simulink model "TST_RailP_VDGradMon"  (R2016b)
settings: Solver=FixedStepDiscrete  StartTime=0.0  StopTime=simTime  FixedStep=sampleTime  RelTol=1e-3
values from neighbouring files (symbols this model uses):
  testCase = 1    [initTST_RailP_VDGradMon_001.m]    (also in initTST_RailP_VDGradMon_002.m = 2; initTST_RailP_VDGradMon_003.m = 3; initTST_RailP_VDGradMon_004.m = 4; initTST_RailP_VDGradMon_005.m = 5)
libraries: simulink x6
settings Model: Creator=wolf072601  LastModifiedBy=wolf072601
settings DebuggingCC: SignalRangeChecking=error

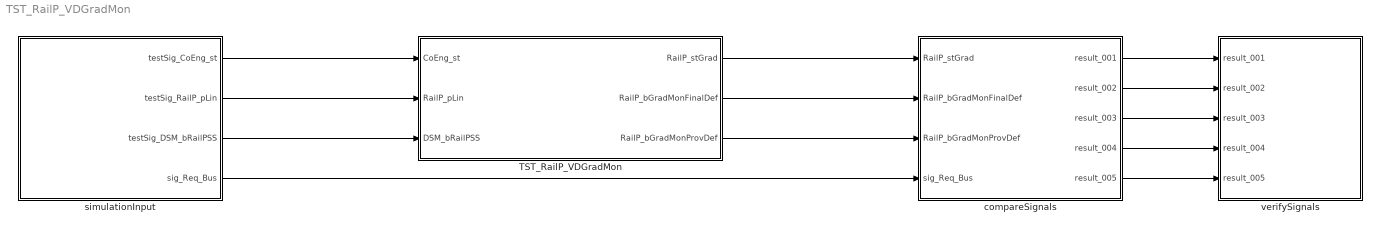
== system TST_RailP_VDGradMon ==
  TST_RailP_VDGradMon : Subsystem
  compareSignals : Subsystem
  simulationInput : Subsystem
  verifySignals : Subsystem
  wires:
  simulationInput/1(testSig_CoEng_st) -> TST_RailP_VDGradMon/1(CoEng_st)
  simulationInput/2(testSig_RailP_pLin) -> TST_RailP_VDGradMon/2(RailP_pLin)
  simulationInput/3(testSig_DSM_bRailPSS) -> TST_RailP_VDGradMon/3(DSM_bRailPSS)
  TST_RailP_VDGradMon/1(RailP_stGrad) -> compareSignals/1(RailP_stGrad)
  TST_RailP_VDGradMon/2(RailP_bGradMonFinalDef) -> compareSignals/2(RailP_bGradMonFinalDef)
  TST_RailP_VDGradMon/3(RailP_bGradMonProvDef) -> compareSignals/3(RailP_bGradMonProvDef)
  simulationInput/4(sig_Req_Bus) -> compareSignals/4(sig_Req_Bus)
  compareSignals/1(result_001) -> verifySignals/1(result_001)
  compareSignals/2(result_002) -> verifySignals/2(result_002)
  compareSignals/3(result_003) -> verifySignals/3(result_003)
  compareSignals/4(result_004) -> verifySignals/4(result_004)
  compareSignals/5(result_005) -> verifySignals/5(result_005)

== system TST_RailP_VDGradMon/TST_RailP_VDGradMon ==
  CoEng_st : Inport
  RailP_pLin : Inport  Port=2
  DSM_bRailPSS : Inport  Port=3
  Function_Call : simulink/Ports & Subsystems/Function-Call Generator  sample_time=sampleTime  numberOfIterations=1
  RailP_VDGradMon : ModelReference  ModelNameDialog=RailP_VDGradMon  ModelReferenceVersion=1.19  TriggerPortName=function  TriggerPortTriggerType=function-call  TriggerPortStatesWhenEnabling=held
  RailP_stGrad : Outport
  RailP_bGradMonFinalDef : Outport  Port=2
  RailP_bGradMonProvDef : Outport  Port=3
  wires:
  Function_Call/1 -> RailP_VDGradMon/Trigger
  CoEng_st/1 -> RailP_VDGradMon/1
  RailP_pLin/1 -> RailP_VDGradMon/2
  DSM_bRailPSS/1 -> RailP_VDGradMon/3
  RailP_VDGradMon/1 -> RailP_stGrad/1
  RailP_VDGradMon/2 -> RailP_bGradMonFinalDef/1
  RailP_VDGradMon/3 -> RailP_bGradMonProvDef/1

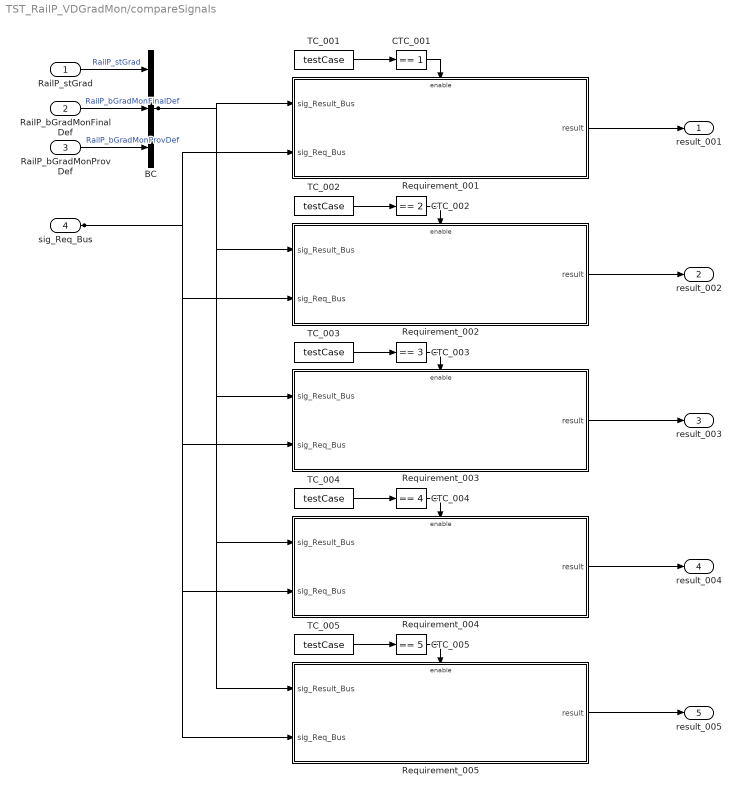
== system TST_RailP_VDGradMon/compareSignals ==
  RailP_stGrad : Inport
  RailP_bGradMonFinalDef : Inport  Port=2
  RailP_bGradMonProvDef : Inport  Port=3
  sig_Req_Bus : Inport  Port=4
  BC : BusCreator  Inputs=3
  CTC_001 : simulink/Logic and Bit Operations/Compare To Constant  relop===  const=1  OutDataTypeStr=boolean
  CTC_002 : simulink/Logic and Bit Operations/Compare To Constant  relop===  const=2  OutDataTypeStr=boolean
  CTC_003 : simulink/Logic and Bit Operations/Compare To Constant  relop===  const=3  OutDataTypeStr=boolean
  CTC_004 : simulink/Logic and Bit Operations/Compare To Constant  relop===  const=4  OutDataTypeStr=boolean
  CTC_005 : simulink/Logic and Bit Operations/Compare To Constant  relop===  const=5  OutDataTypeStr=boolean
  Requirement_001 : Subsystem
  Requirement_002 : Subsystem
  Requirement_003 : Subsystem
  Requirement_004 : Subsystem
  Requirement_005 : Subsystem
  TC_001 : Constant  Value=testCase
  TC_002 : Constant  Value=testCase
  TC_003 : Constant  Value=testCase
  TC_004 : Constant  Value=testCase
  TC_005 : Constant  Value=testCase
  result_001 : Outport
  result_002 : Outport  Port=2
  result_003 : Outport  Port=3
  result_004 : Outport  Port=4
  result_005 : Outport  Port=5
  wires:
  RailP_stGrad/1 -> BC/1  "RailP_stGrad"
  RailP_bGradMonFinalDef/1 -> BC/2  "RailP_bGradMonFinalDef"
  RailP_bGradMonProvDef/1 -> BC/3  "RailP_bGradMonProvDef"
  TC_001/1 -> CTC_001/1
  CTC_001/1 -> Requirement_001/Enable
  sig_Req_Bus/1 -> Requirement_001/2(sig_Req_Bus), Requirement_002/2(sig_Req_Bus), Requirement_003/2(sig_Req_Bus), Requirement_004/2(sig_Req_Bus), Requirement_005/2(sig_Req_Bus)
  BC/1 -> Requirement_001/1(sig_Result_Bus), Requirement_002/1(sig_Result_Bus), Requirement_003/1(sig_Result_Bus), Requirement_004/1(sig_Result_Bus), Requirement_005/1(sig_Result_Bus)
  Requirement_001/1(result) -> result_001/1
  TC_002/1 -> CTC_002/1
  CTC_002/1 -> Requirement_002/Enable
  Requirement_002/1(result) -> result_002/1
  TC_003/1 -> CTC_003/1
  CTC_003/1 -> Requirement_003/Enable
  Requirement_003/1(result) -> result_003/1
  TC_004/1 -> CTC_004/1
  CTC_004/1 -> Requirement_004/Enable
  Requirement_004/1(result) -> result_004/1
  TC_005/1 -> CTC_005/1
  CTC_005/1 -> Requirement_005/Enable
  Requirement_005/1(result) -> result_005/1

== system TST_RailP_VDGradMon/simulationInput ==
  BS : BusSelector  OutputSignals=testSig_CoEng_st,testSig_RailP_pLin,testSig_DSM_bRailPSS
  MPSw : MultiPortSwitch  Inputs=5  SaturateOnIntegerOverflow=on  InputSameDT=on
  TestCase : Constant  Value=testCase
  testSignals_R001 : Subsystem
  testSignals_R002 : Subsystem
  testSignals_R003 : Subsystem
  testSignals_R004 : Subsystem
  testSignals_R005 : Subsystem
  testSig_CoEng_st : Outport
  testSig_RailP_pLin : Outport  Port=2
  testSig_DSM_bRailPSS : Outport  Port=3
  sig_Req_Bus : Outport  Port=4
  wires:
  BS/1 -> testSig_CoEng_st/1  "<testSig_CoEng_st>"
  BS/2 -> testSig_RailP_pLin/1  "<testSig_RailP_pLin>"
  BS/3 -> testSig_DSM_bRailPSS/1  "<testSig_DSM_bRailPSS>"
  MPSw/1 -> BS/1, sig_Req_Bus/1
  TestCase/1 -> MPSw/1
  testSignals_R001/1(testSignals) -> MPSw/2
  testSignals_R002/1(testSignals) -> MPSw/3
  testSignals_R003/1(testSignals) -> MPSw/4
  testSignals_R004/1(testSignals) -> MPSw/5
  testSignals_R005/1(testSignals) -> MPSw/6

== system TST_RailP_VDGradMon/verifySignals ==
  result_001 : Inport
  result_002 : Inport  Port=2
  result_003 : Inport  Port=3
  result_004 : Inport  Port=4
  result_005 : Inport  Port=5
  Assertion_001 : Assertion  Enabled=off
  Assertion_002 : Assertion  Enabled=off
  Assertion_003 : Assertion  Enabled=off
  Assertion_004 : Assertion  Enabled=off
  Assertion_005 : Assertion  Enabled=off
  wires:
  result_001/1 -> Assertion_001/1
  result_002/1 -> Assertion_002/1
  result_003/1 -> Assertion_003/1
  result_004/1 -> Assertion_004/1
  result_005/1 -> Assertion_005/1

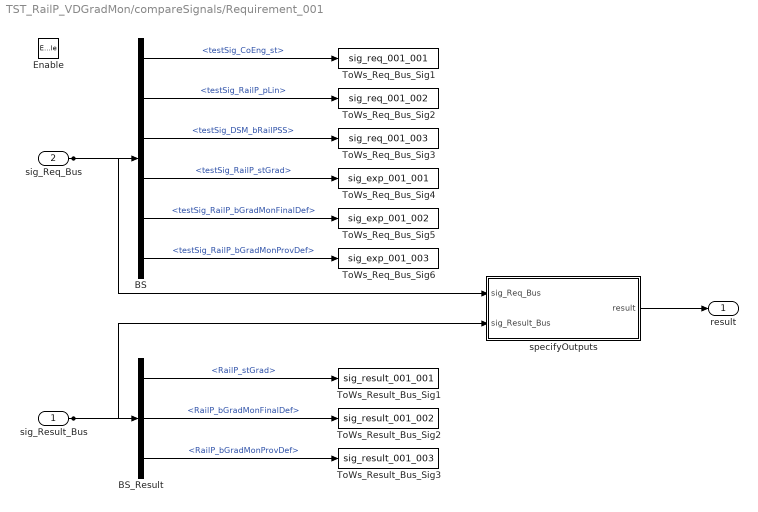
== system TST_RailP_VDGradMon/compareSignals/Requirement_001 ==
  sig_Result_Bus : Inport
  sig_Req_Bus : Inport  Port=2
  Enable : EnablePort
  BS : BusSelector  OutputSignals=testSig_CoEng_st,testSig_RailP_pLin,testSig_DSM_bRailPSS,testSig_RailP_stGrad,testSig_RailP_bGradMonFinalDef,testSig_RailP_bGradMonProvDef
  BS_Result : BusSelector  OutputSignals=RailP_stGrad,RailP_bGradMonFinalDef,RailP_bGradMonProvDef
  ToWs_Req_Bus_Sig1 : ToWorkspace  VariableName=sig_req_001_001  SaveFormat=Structure With Time
  ToWs_Req_Bus_Sig2 : ToWorkspace  VariableName=sig_req_001_002  SaveFormat=Structure With Time
  ToWs_Req_Bus_Sig3 : ToWorkspace  VariableName=sig_req_001_003  SaveFormat=Structure With Time
  ToWs_Req_Bus_Sig4 : ToWorkspace  VariableName=sig_exp_001_001  SaveFormat=Structure With Time
  ToWs_Req_Bus_Sig5 : ToWorkspace  VariableName=sig_exp_001_002  SaveFormat=Structure With Time
  ToWs_Req_Bus_Sig6 : ToWorkspace  VariableName=sig_exp_001_003  SaveFormat=Structure With Time
  ToWs_Result_Bus_Sig1 : ToWorkspace  VariableName=sig_result_001_001  SaveFormat=Structure With Time
  ToWs_Result_Bus_Sig2 : ToWorkspace  VariableName=sig_result_001_002  SaveFormat=Structure With Time
  ToWs_Result_Bus_Sig3 : ToWorkspace  VariableName=sig_result_001_003  SaveFormat=Structure With Time
  specifyOutputs : Subsystem
  result : Outport
  wires:
  sig_Req_Bus/1 -> BS/1, specifyOutputs/1(sig_Req_Bus)
  BS/1 -> ToWs_Req_Bus_Sig1/1  "<testSig_CoEng_st>"
  BS/2 -> ToWs_Req_Bus_Sig2/1  "<testSig_RailP_pLin>"
  BS/3 -> ToWs_Req_Bus_Sig3/1  "<testSig_DSM_bRailPSS>"
  BS/4 -> ToWs_Req_Bus_Sig4/1  "<testSig_RailP_stGrad>"
  BS/5 -> ToWs_Req_Bus_Sig5/1  "<testSig_RailP_bGradMonFinalDef>"
  BS/6 -> ToWs_Req_Bus_Sig6/1  "<testSig_RailP_bGradMonProvDef>"
  sig_Result_Bus/1 -> BS_Result/1, specifyOutputs/2(sig_Result_Bus)
  BS_Result/1 -> ToWs_Result_Bus_Sig1/1  "<RailP_stGrad>"
  BS_Result/2 -> ToWs_Result_Bus_Sig2/1  "<RailP_bGradMonFinalDef>"
  BS_Result/3 -> ToWs_Result_Bus_Sig3/1  "<RailP_bGradMonProvDef>"
  specifyOutputs/1(result) -> result/1

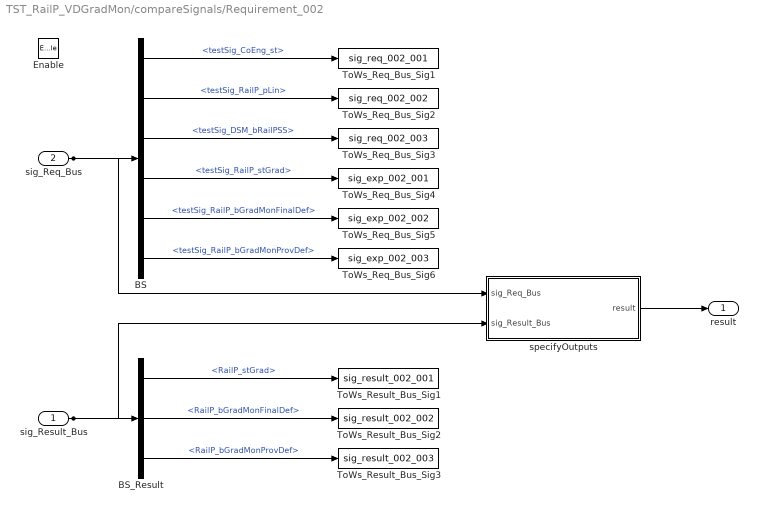
== system TST_RailP_VDGradMon/compareSignals/Requirement_002 ==
  sig_Result_Bus : Inport
  sig_Req_Bus : Inport  Port=2
  Enable : EnablePort
  BS : BusSelector  OutputSignals=testSig_CoEng_st,testSig_RailP_pLin,testSig_DSM_bRailPSS,testSig_RailP_stGrad,testSig_RailP_bGradMonFinalDef,testSig_RailP_bGradMonProvDef
  BS_Result : BusSelector  OutputSignals=RailP_stGrad,RailP_bGradMonFinalDef,RailP_bGradMonProvDef
  ToWs_Req_Bus_Sig1 : ToWorkspace  VariableName=sig_req_002_001  SaveFormat=Structure With Time
  ToWs_Req_Bus_Sig2 : ToWorkspace  VariableName=sig_req_002_002  SaveFormat=Structure With Time
  ToWs_Req_Bus_Sig3 : ToWorkspace  VariableName=sig_req_002_003  SaveFormat=Structure With Time
  ToWs_Req_Bus_Sig4 : ToWorkspace  VariableName=sig_exp_002_001  SaveFormat=Structure With Time
  ToWs_Req_Bus_Sig5 : ToWorkspace  VariableName=sig_exp_002_002  SaveFormat=Structure With Time
  ToWs_Req_Bus_Sig6 : ToWorkspace  VariableName=sig_exp_002_003  SaveFormat=Structure With Time
  ToWs_Result_Bus_Sig1 : ToWorkspace  VariableName=sig_result_002_001  SaveFormat=Structure With Time
  ToWs_Result_Bus_Sig2 : ToWorkspace  VariableName=sig_result_002_002  SaveFormat=Structure With Time
  ToWs_Result_Bus_Sig3 : ToWorkspace  VariableName=sig_result_002_003  SaveFormat=Structure With Time
  specifyOutputs : Subsystem
  result : Outport
  wires:
  sig_Req_Bus/1 -> BS/1, specifyOutputs/1(sig_Req_Bus)
  BS/1 -> ToWs_Req_Bus_Sig1/1  "<testSig_CoEng_st>"
  BS/2 -> ToWs_Req_Bus_Sig2/1  "<testSig_RailP_pLin>"
  BS/3 -> ToWs_Req_Bus_Sig3/1  "<testSig_DSM_bRailPSS>"
  BS/4 -> ToWs_Req_Bus_Sig4/1  "<testSig_RailP_stGrad>"
  BS/5 -> ToWs_Req_Bus_Sig5/1  "<testSig_RailP_bGradMonFinalDef>"
  BS/6 -> ToWs_Req_Bus_Sig6/1  "<testSig_RailP_bGradMonProvDef>"
  sig_Result_Bus/1 -> BS_Result/1, specifyOutputs/2(sig_Result_Bus)
  BS_Result/1 -> ToWs_Result_Bus_Sig1/1  "<RailP_stGrad>"
  BS_Result/2 -> ToWs_Result_Bus_Sig2/1  "<RailP_bGradMonFinalDef>"
  BS_Result/3 -> ToWs_Result_Bus_Sig3/1  "<RailP_bGradMonProvDef>"
  specifyOutputs/1(result) -> result/1

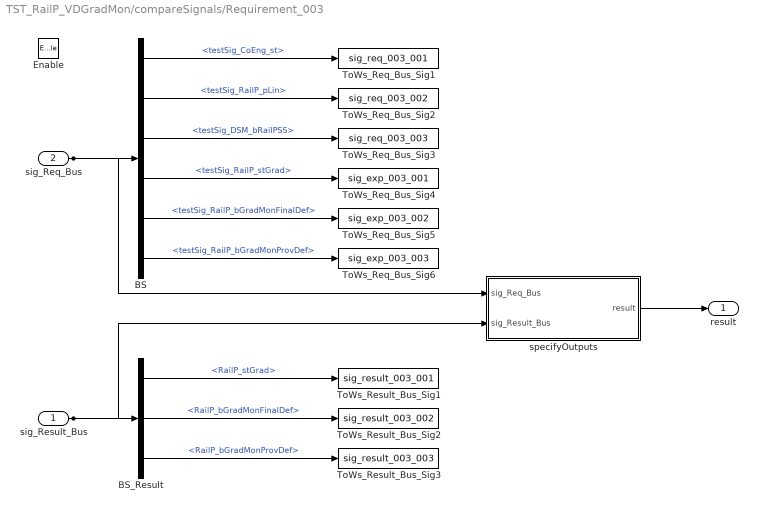
== system TST_RailP_VDGradMon/compareSignals/Requirement_003 ==
  sig_Result_Bus : Inport
  sig_Req_Bus : Inport  Port=2
  Enable : EnablePort
  BS : BusSelector  OutputSignals=testSig_CoEng_st,testSig_RailP_pLin,testSig_DSM_bRailPSS,testSig_RailP_stGrad,testSig_RailP_bGradMonFinalDef,testSig_RailP_bGradMonProvDef
  BS_Result : BusSelector  OutputSignals=RailP_stGrad,RailP_bGradMonFinalDef,RailP_bGradMonProvDef
  ToWs_Req_Bus_Sig1 : ToWorkspace  VariableName=sig_req_003_001  SaveFormat=Structure With Time
  ToWs_Req_Bus_Sig2 : ToWorkspace  VariableName=sig_req_003_002  SaveFormat=Structure With Time
  ToWs_Req_Bus_Sig3 : ToWorkspace  VariableName=sig_req_003_003  SaveFormat=Structure With Time
  ToWs_Req_Bus_Sig4 : ToWorkspace  VariableName=sig_exp_003_001  SaveFormat=Structure With Time
  ToWs_Req_Bus_Sig5 : ToWorkspace  VariableName=sig_exp_003_002  SaveFormat=Structure With Time
  ToWs_Req_Bus_Sig6 : ToWorkspace  VariableName=sig_exp_003_003  SaveFormat=Structure With Time
  ToWs_Result_Bus_Sig1 : ToWorkspace  VariableName=sig_result_003_001  SaveFormat=Structure With Time
  ToWs_Result_Bus_Sig2 : ToWorkspace  VariableName=sig_result_003_002  SaveFormat=Structure With Time
  ToWs_Result_Bus_Sig3 : ToWorkspace  VariableName=sig_result_003_003  SaveFormat=Structure With Time
  specifyOutputs : Subsystem
  result : Outport
  wires:
  sig_Req_Bus/1 -> BS/1, specifyOutputs/1(sig_Req_Bus)
  BS/1 -> ToWs_Req_Bus_Sig1/1  "<testSig_CoEng_st>"
  BS/2 -> ToWs_Req_Bus_Sig2/1  "<testSig_RailP_pLin>"
  BS/3 -> ToWs_Req_Bus_Sig3/1  "<testSig_DSM_bRailPSS>"
  BS/4 -> ToWs_Req_Bus_Sig4/1  "<testSig_RailP_stGrad>"
  BS/5 -> ToWs_Req_Bus_Sig5/1  "<testSig_RailP_bGradMonFinalDef>"
  BS/6 -> ToWs_Req_Bus_Sig6/1  "<testSig_RailP_bGradMonProvDef>"
  sig_Result_Bus/1 -> BS_Result/1, specifyOutputs/2(sig_Result_Bus)
  BS_Result/1 -> ToWs_Result_Bus_Sig1/1  "<RailP_stGrad>"
  BS_Result/2 -> ToWs_Result_Bus_Sig2/1  "<RailP_bGradMonFinalDef>"
  BS_Result/3 -> ToWs_Result_Bus_Sig3/1  "<RailP_bGradMonProvDef>"
  specifyOutputs/1(result) -> result/1

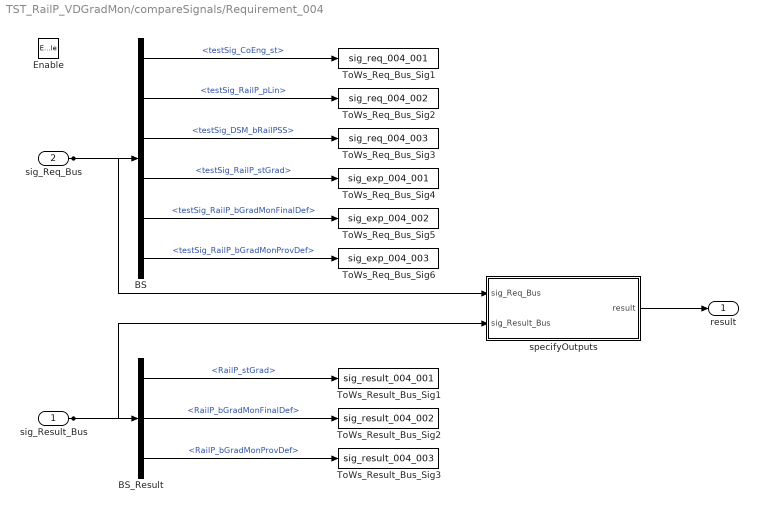
== system TST_RailP_VDGradMon/compareSignals/Requirement_004 ==
  sig_Result_Bus : Inport
  sig_Req_Bus : Inport  Port=2
  Enable : EnablePort
  BS : BusSelector  OutputSignals=testSig_CoEng_st,testSig_RailP_pLin,testSig_DSM_bRailPSS,testSig_RailP_stGrad,testSig_RailP_bGradMonFinalDef,testSig_RailP_bGradMonProvDef
  BS_Result : BusSelector  OutputSignals=RailP_stGrad,RailP_bGradMonFinalDef,RailP_bGradMonProvDef
  ToWs_Req_Bus_Sig1 : ToWorkspace  VariableName=sig_req_004_001  SaveFormat=Structure With Time
  ToWs_Req_Bus_Sig2 : ToWorkspace  VariableName=sig_req_004_002  SaveFormat=Structure With Time
  ToWs_Req_Bus_Sig3 : ToWorkspace  VariableName=sig_req_004_003  SaveFormat=Structure With Time
  ToWs_Req_Bus_Sig4 : ToWorkspace  VariableName=sig_exp_004_001  SaveFormat=Structure With Time
  ToWs_Req_Bus_Sig5 : ToWorkspace  VariableName=sig_exp_004_002  SaveFormat=Structure With Time
  ToWs_Req_Bus_Sig6 : ToWorkspace  VariableName=sig_exp_004_003  SaveFormat=Structure With Time
  ToWs_Result_Bus_Sig1 : ToWorkspace  VariableName=sig_result_004_001  SaveFormat=Structure With Time
  ToWs_Result_Bus_Sig2 : ToWorkspace  VariableName=sig_result_004_002  SaveFormat=Structure With Time
  ToWs_Result_Bus_Sig3 : ToWorkspace  VariableName=sig_result_004_003  SaveFormat=Structure With Time
  specifyOutputs : Subsystem
  result : Outport
  wires:
  sig_Req_Bus/1 -> BS/1, specifyOutputs/1(sig_Req_Bus)
  BS/1 -> ToWs_Req_Bus_Sig1/1  "<testSig_CoEng_st>"
  BS/2 -> ToWs_Req_Bus_Sig2/1  "<testSig_RailP_pLin>"
  BS/3 -> ToWs_Req_Bus_Sig3/1  "<testSig_DSM_bRailPSS>"
  BS/4 -> ToWs_Req_Bus_Sig4/1  "<testSig_RailP_stGrad>"
  BS/5 -> ToWs_Req_Bus_Sig5/1  "<testSig_RailP_bGradMonFinalDef>"
  BS/6 -> ToWs_Req_Bus_Sig6/1  "<testSig_RailP_bGradMonProvDef>"
  sig_Result_Bus/1 -> BS_Result/1, specifyOutputs/2(sig_Result_Bus)
  BS_Result/1 -> ToWs_Result_Bus_Sig1/1  "<RailP_stGrad>"
  BS_Result/2 -> ToWs_Result_Bus_Sig2/1  "<RailP_bGradMonFinalDef>"
  BS_Result/3 -> ToWs_Result_Bus_Sig3/1  "<RailP_bGradMonProvDef>"
  specifyOutputs/1(result) -> result/1

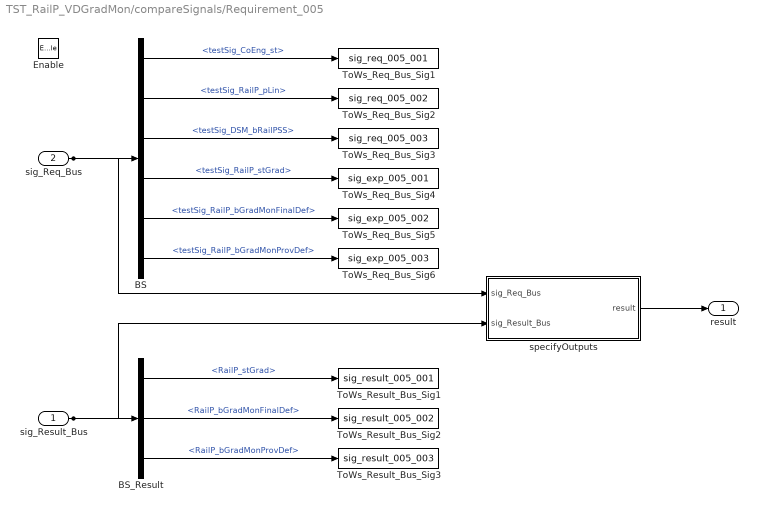
== system TST_RailP_VDGradMon/compareSignals/Requirement_005 ==
  sig_Result_Bus : Inport
  sig_Req_Bus : Inport  Port=2
  Enable : EnablePort
  BS : BusSelector  OutputSignals=testSig_CoEng_st,testSig_RailP_pLin,testSig_DSM_bRailPSS,testSig_RailP_stGrad,testSig_RailP_bGradMonFinalDef,testSig_RailP_bGradMonProvDef
  BS_Result : BusSelector  OutputSignals=RailP_stGrad,RailP_bGradMonFinalDef,RailP_bGradMonProvDef
  ToWs_Req_Bus_Sig1 : ToWorkspace  VariableName=sig_req_005_001  SaveFormat=Structure With Time
  ToWs_Req_Bus_Sig2 : ToWorkspace  VariableName=sig_req_005_002  SaveFormat=Structure With Time
  ToWs_Req_Bus_Sig3 : ToWorkspace  VariableName=sig_req_005_003  SaveFormat=Structure With Time
  ToWs_Req_Bus_Sig4 : ToWorkspace  VariableName=sig_exp_005_001  SaveFormat=Structure With Time
  ToWs_Req_Bus_Sig5 : ToWorkspace  VariableName=sig_exp_005_002  SaveFormat=Structure With Time
  ToWs_Req_Bus_Sig6 : ToWorkspace  VariableName=sig_exp_005_003  SaveFormat=Structure With Time
  ToWs_Result_Bus_Sig1 : ToWorkspace  VariableName=sig_result_005_001  SaveFormat=Structure With Time
  ToWs_Result_Bus_Sig2 : ToWorkspace  VariableName=sig_result_005_002  SaveFormat=Structure With Time
  ToWs_Result_Bus_Sig3 : ToWorkspace  VariableName=sig_result_005_003  SaveFormat=Structure With Time
  specifyOutputs : Subsystem
  result : Outport
  wires:
  sig_Req_Bus/1 -> BS/1, specifyOutputs/1(sig_Req_Bus)
  BS/1 -> ToWs_Req_Bus_Sig1/1  "<testSig_CoEng_st>"
  BS/2 -> ToWs_Req_Bus_Sig2/1  "<testSig_RailP_pLin>"
  BS/3 -> ToWs_Req_Bus_Sig3/1  "<testSig_DSM_bRailPSS>"
  BS/4 -> ToWs_Req_Bus_Sig4/1  "<testSig_RailP_stGrad>"
  BS/5 -> ToWs_Req_Bus_Sig5/1  "<testSig_RailP_bGradMonFinalDef>"
  BS/6 -> ToWs_Req_Bus_Sig6/1  "<testSig_RailP_bGradMonProvDef>"
  sig_Result_Bus/1 -> BS_Result/1, specifyOutputs/2(sig_Result_Bus)
  BS_Result/1 -> ToWs_Result_Bus_Sig1/1  "<RailP_stGrad>"
  BS_Result/2 -> ToWs_Result_Bus_Sig2/1  "<RailP_bGradMonFinalDef>"
  BS_Result/3 -> ToWs_Result_Bus_Sig3/1  "<RailP_bGradMonProvDef>"
  specifyOutputs/1(result) -> result/1

== system TST_RailP_VDGradMon/simulationInput/testSignals_R001 ==
  BC : BusCreator  Inputs=6
  spec_CoEng_st : FromWorkspace  VariableName=testSig_CoEng_st  Interpolate=off  OutputAfterFinalValue=Holding final value
  spec_DSM_bRailPSS : FromWorkspace  VariableName=testSig_DSM_bRailPSS  Interpolate=off  OutputAfterFinalValue=Holding final value
  spec_RailP_bGradMonFinalDef : FromWorkspace  VariableName=testSig_RailP_bGradMonFinalDef  Interpolate=off  OutputAfterFinalValue=Holding final value
  spec_RailP_bGradMonProvDef : FromWorkspace  VariableName=testSig_RailP_bGradMonProvDef  Interpolate=off  OutputAfterFinalValue=Holding final value
  spec_RailP_pLin : FromWorkspace  VariableName=testSig_RailP_pLin  Interpolate=off  OutputAfterFinalValue=Holding final value
  spec_RailP_stGrad : FromWorkspace  VariableName=testSig_RailP_stGrad  Interpolate=off  OutputAfterFinalValue=Holding final value
  testSignals : Outport
  wires:
  BC/1 -> testSignals/1
  spec_CoEng_st/1 -> BC/1  "testSig_CoEng_st"
  spec_RailP_pLin/1 -> BC/2  "testSig_RailP_pLin"
  spec_DSM_bRailPSS/1 -> BC/3  "testSig_DSM_bRailPSS"
  spec_RailP_stGrad/1 -> BC/4  "testSig_RailP_stGrad"
  spec_RailP_bGradMonFinalDef/1 -> BC/5  "testSig_RailP_bGradMonFinalDef"
  spec_RailP_bGradMonProvDef/1 -> BC/6  "testSig_RailP_bGradMonProvDef"

== system TST_RailP_VDGradMon/simulationInput/testSignals_R002 ==
  BC : BusCreator  Inputs=6
  spec_CoEng_st : FromWorkspace  VariableName=testSig_CoEng_st  Interpolate=off  OutputAfterFinalValue=Holding final value
  spec_DSM_bRailPSS : FromWorkspace  VariableName=testSig_DSM_bRailPSS  Interpolate=off  OutputAfterFinalValue=Holding final value
  spec_RailP_bGradMonFinalDef : FromWorkspace  VariableName=testSig_RailP_bGradMonFinalDef  Interpolate=off  OutputAfterFinalValue=Holding final value
  spec_RailP_bGradMonProvDef : FromWorkspace  VariableName=testSig_RailP_bGradMonProvDef  Interpolate=off  OutputAfterFinalValue=Holding final value
  spec_RailP_pLin : FromWorkspace  VariableName=testSig_RailP_pLin  Interpolate=off  OutputAfterFinalValue=Holding final value
  spec_RailP_stGrad : FromWorkspace  VariableName=testSig_RailP_stGrad  Interpolate=off  OutputAfterFinalValue=Holding final value
  testSignals : Outport
  wires:
  BC/1 -> testSignals/1
  spec_CoEng_st/1 -> BC/1  "testSig_CoEng_st"
  spec_RailP_pLin/1 -> BC/2  "testSig_RailP_pLin"
  spec_DSM_bRailPSS/1 -> BC/3  "testSig_DSM_bRailPSS"
  spec_RailP_stGrad/1 -> BC/4  "testSig_RailP_stGrad"
  spec_RailP_bGradMonFinalDef/1 -> BC/5  "testSig_RailP_bGradMonFinalDef"
  spec_RailP_bGradMonProvDef/1 -> BC/6  "testSig_RailP_bGradMonProvDef"

== system TST_RailP_VDGradMon/simulationInput/testSignals_R003 ==
  BC : BusCreator  Inputs=6
  spec_CoEng_st : FromWorkspace  VariableName=testSig_CoEng_st  Interpolate=off  OutputAfterFinalValue=Holding final value
  spec_DSM_bRailPSS : FromWorkspace  VariableName=testSig_DSM_bRailPSS  Interpolate=off  OutputAfterFinalValue=Holding final value
  spec_RailP_bGradMonFinalDef : FromWorkspace  VariableName=testSig_RailP_bGradMonFinalDef  Interpolate=off  OutputAfterFinalValue=Holding final value
  spec_RailP_bGradMonProvDef : FromWorkspace  VariableName=testSig_RailP_bGradMonProvDef  Interpolate=off  OutputAfterFinalValue=Holding final value
  spec_RailP_pLin : FromWorkspace  VariableName=testSig_RailP_pLin  Interpolate=off  OutputAfterFinalValue=Holding final value
  spec_RailP_stGrad : FromWorkspace  VariableName=testSig_RailP_stGrad  Interpolate=off  OutputAfterFinalValue=Holding final value
  testSignals : Outport
  wires:
  BC/1 -> testSignals/1
  spec_CoEng_st/1 -> BC/1  "testSig_CoEng_st"
  spec_RailP_pLin/1 -> BC/2  "testSig_RailP_pLin"
  spec_DSM_bRailPSS/1 -> BC/3  "testSig_DSM_bRailPSS"
  spec_RailP_stGrad/1 -> BC/4  "testSig_RailP_stGrad"
  spec_RailP_bGradMonFinalDef/1 -> BC/5  "testSig_RailP_bGradMonFinalDef"
  spec_RailP_bGradMonProvDef/1 -> BC/6  "testSig_RailP_bGradMonProvDef"

== system TST_RailP_VDGradMon/simulationInput/testSignals_R004 ==
  BC : BusCreator  Inputs=6
  spec_CoEng_st : FromWorkspace  VariableName=testSig_CoEng_st  Interpolate=off  OutputAfterFinalValue=Holding final value
  spec_DSM_bRailPSS : FromWorkspace  VariableName=testSig_DSM_bRailPSS  Interpolate=off  OutputAfterFinalValue=Holding final value
  spec_RailP_bGradMonFinalDef : FromWorkspace  VariableName=testSig_RailP_bGradMonFinalDef  Interpolate=off  OutputAfterFinalValue=Holding final value
  spec_RailP_bGradMonProvDef : FromWorkspace  VariableName=testSig_RailP_bGradMonProvDef  Interpolate=off  OutputAfterFinalValue=Holding final value
  spec_RailP_pLin : FromWorkspace  VariableName=testSig_RailP_pLin  Interpolate=off  OutputAfterFinalValue=Holding final value
  spec_RailP_stGrad : FromWorkspace  VariableName=testSig_RailP_stGrad  Interpolate=off  OutputAfterFinalValue=Holding final value
  testSignals : Outport
  wires:
  BC/1 -> testSignals/1
  spec_CoEng_st/1 -> BC/1  "testSig_CoEng_st"
  spec_RailP_pLin/1 -> BC/2  "testSig_RailP_pLin"
  spec_DSM_bRailPSS/1 -> BC/3  "testSig_DSM_bRailPSS"
  spec_RailP_stGrad/1 -> BC/4  "testSig_RailP_stGrad"
  spec_RailP_bGradMonFinalDef/1 -> BC/5  "testSig_RailP_bGradMonFinalDef"
  spec_RailP_bGradMonProvDef/1 -> BC/6  "testSig_RailP_bGradMonProvDef"

== system TST_RailP_VDGradMon/simulationInput/testSignals_R005 ==
  BC : BusCreator  Inputs=6
  spec_CoEng_st : FromWorkspace  VariableName=testSig_CoEng_st  Interpolate=off  OutputAfterFinalValue=Holding final value
  spec_DSM_bRailPSS : FromWorkspace  VariableName=testSig_DSM_bRailPSS  Interpolate=off  OutputAfterFinalValue=Holding final value
  spec_RailP_bGradMonFinalDef : FromWorkspace  VariableName=testSig_RailP_bGradMonFinalDef  Interpolate=off  OutputAfterFinalValue=Holding final value
  spec_RailP_bGradMonProvDef : FromWorkspace  VariableName=testSig_RailP_bGradMonProvDef  Interpolate=off  OutputAfterFinalValue=Holding final value
  spec_RailP_pLin : FromWorkspace  VariableName=testSig_RailP_pLin  Interpolate=off  OutputAfterFinalValue=Holding final value
  spec_RailP_stGrad : FromWorkspace  VariableName=testSig_RailP_stGrad  Interpolate=off  OutputAfterFinalValue=Holding final value
  testSignals : Outport
  wires:
  BC/1 -> testSignals/1
  spec_CoEng_st/1 -> BC/1  "testSig_CoEng_st"
  spec_RailP_pLin/1 -> BC/2  "testSig_RailP_pLin"
  spec_DSM_bRailPSS/1 -> BC/3  "testSig_DSM_bRailPSS"
  spec_RailP_stGrad/1 -> BC/4  "testSig_RailP_stGrad"
  spec_RailP_bGradMonFinalDef/1 -> BC/5  "testSig_RailP_bGradMonFinalDef"
  spec_RailP_bGradMonProvDef/1 -> BC/6  "testSig_RailP_bGradMonProvDef"

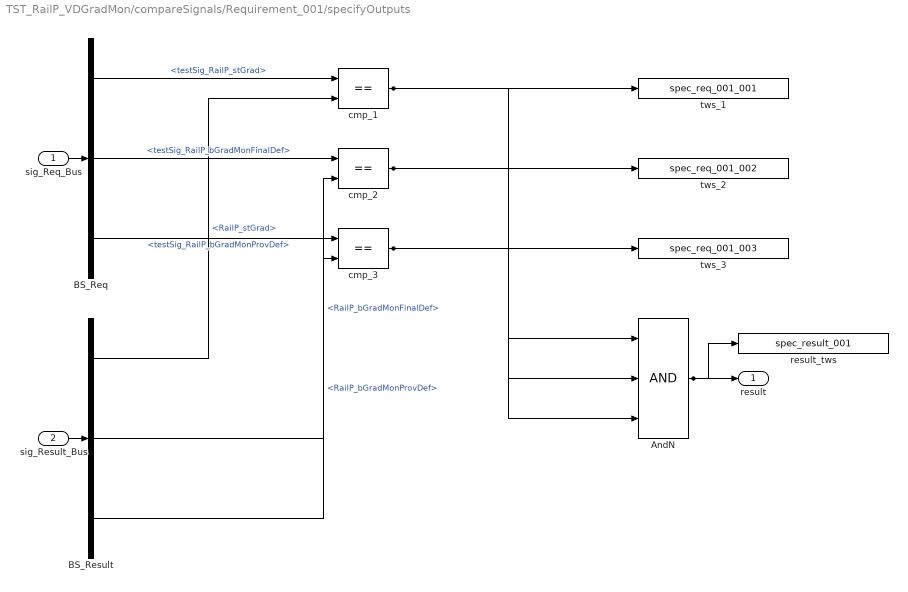
== system TST_RailP_VDGradMon/compareSignals/Requirement_001/specifyOutputs ==
  sig_Req_Bus : Inport
  sig_Result_Bus : Inport  Port=2
  AndN : Logic  Inputs=3
  BS_Req : BusSelector  OutputSignals=testSig_RailP_stGrad,testSig_RailP_bGradMonFinalDef,testSig_RailP_bGradMonProvDef
  BS_Result : BusSelector  OutputSignals=RailP_stGrad,RailP_bGradMonFinalDef,RailP_bGradMonProvDef
  cmp_1 : RelationalOperator  Operator===  RndMeth=Nearest  InputSameDT=on
  cmp_2 : RelationalOperator  Operator===  RndMeth=Nearest  InputSameDT=on
  cmp_3 : RelationalOperator  Operator===  RndMeth=Nearest  InputSameDT=on
  result_tws : ToWorkspace  VariableName=spec_result_001
  tws_1 : ToWorkspace  VariableName=spec_req_001_001
  tws_2 : ToWorkspace  VariableName=spec_req_001_002
  tws_3 : ToWorkspace  VariableName=spec_req_001_003
  result : Outport
  wires:
  sig_Req_Bus/1 -> BS_Req/1
  sig_Result_Bus/1 -> BS_Result/1
  AndN/1 -> result/1, result_tws/1
  BS_Req/1 -> cmp_1/1  "<testSig_RailP_stGrad>"
  BS_Result/1 -> cmp_1/2  "<RailP_stGrad>"
  cmp_1/1 -> tws_1/1, AndN/1
  BS_Req/2 -> cmp_2/1  "<testSig_RailP_bGradMonFinalDef>"
  BS_Result/2 -> cmp_2/2  "<RailP_bGradMonFinalDef>"
  cmp_2/1 -> tws_2/1, AndN/2
  BS_Req/3 -> cmp_3/1  "<testSig_RailP_bGradMonProvDef>"
  BS_Result/3 -> cmp_3/2  "<RailP_bGradMonProvDef>"
  cmp_3/1 -> tws_3/1, AndN/3

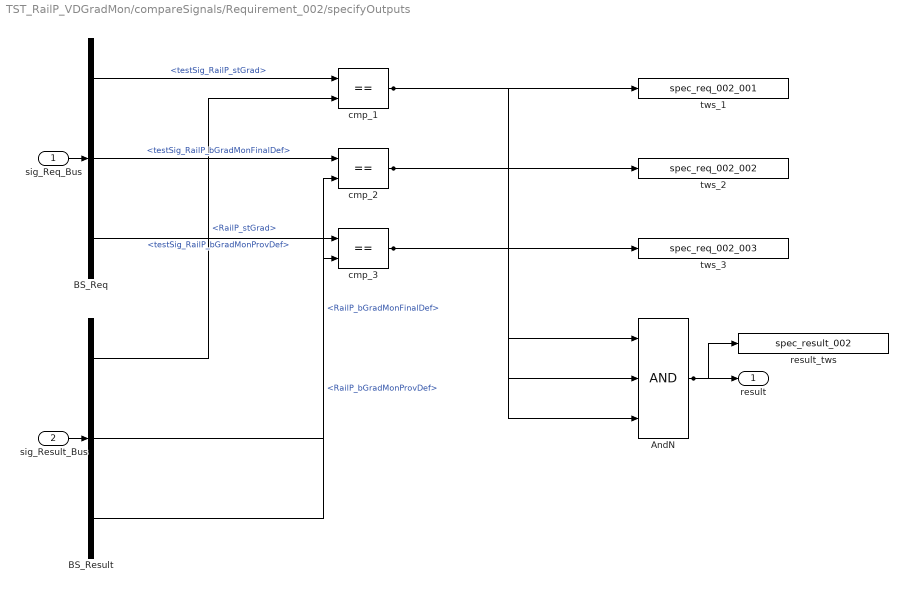
== system TST_RailP_VDGradMon/compareSignals/Requirement_002/specifyOutputs ==
  sig_Req_Bus : Inport
  sig_Result_Bus : Inport  Port=2
  AndN : Logic  Inputs=3
  BS_Req : BusSelector  OutputSignals=testSig_RailP_stGrad,testSig_RailP_bGradMonFinalDef,testSig_RailP_bGradMonProvDef
  BS_Result : BusSelector  OutputSignals=RailP_stGrad,RailP_bGradMonFinalDef,RailP_bGradMonProvDef
  cmp_1 : RelationalOperator  Operator===  RndMeth=Nearest  InputSameDT=on
  cmp_2 : RelationalOperator  Operator===  RndMeth=Nearest  InputSameDT=on
  cmp_3 : RelationalOperator  Operator===  RndMeth=Nearest  InputSameDT=on
  result_tws : ToWorkspace  VariableName=spec_result_002
  tws_1 : ToWorkspace  VariableName=spec_req_002_001
  tws_2 : ToWorkspace  VariableName=spec_req_002_002
  tws_3 : ToWorkspace  VariableName=spec_req_002_003
  result : Outport
  wires:
  sig_Req_Bus/1 -> BS_Req/1
  sig_Result_Bus/1 -> BS_Result/1
  AndN/1 -> result/1, result_tws/1
  BS_Req/1 -> cmp_1/1  "<testSig_RailP_stGrad>"
  BS_Result/1 -> cmp_1/2  "<RailP_stGrad>"
  cmp_1/1 -> tws_1/1, AndN/1
  BS_Req/2 -> cmp_2/1  "<testSig_RailP_bGradMonFinalDef>"
  BS_Result/2 -> cmp_2/2  "<RailP_bGradMonFinalDef>"
  cmp_2/1 -> tws_2/1, AndN/2
  BS_Req/3 -> cmp_3/1  "<testSig_RailP_bGradMonProvDef>"
  BS_Result/3 -> cmp_3/2  "<RailP_bGradMonProvDef>"
  cmp_3/1 -> tws_3/1, AndN/3

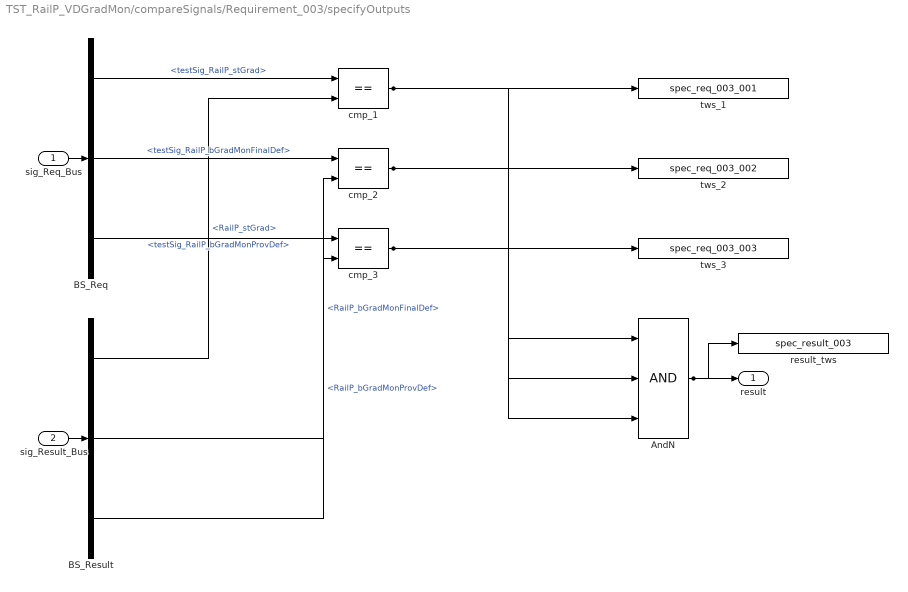
== system TST_RailP_VDGradMon/compareSignals/Requirement_003/specifyOutputs ==
  sig_Req_Bus : Inport
  sig_Result_Bus : Inport  Port=2
  AndN : Logic  Inputs=3
  BS_Req : BusSelector  OutputSignals=testSig_RailP_stGrad,testSig_RailP_bGradMonFinalDef,testSig_RailP_bGradMonProvDef
  BS_Result : BusSelector  OutputSignals=RailP_stGrad,RailP_bGradMonFinalDef,RailP_bGradMonProvDef
  cmp_1 : RelationalOperator  Operator===  RndMeth=Nearest  InputSameDT=on
  cmp_2 : RelationalOperator  Operator===  RndMeth=Nearest  InputSameDT=on
  cmp_3 : RelationalOperator  Operator===  RndMeth=Nearest  InputSameDT=on
  result_tws : ToWorkspace  VariableName=spec_result_003
  tws_1 : ToWorkspace  VariableName=spec_req_003_001
  tws_2 : ToWorkspace  VariableName=spec_req_003_002
  tws_3 : ToWorkspace  VariableName=spec_req_003_003
  result : Outport
  wires:
  sig_Req_Bus/1 -> BS_Req/1
  sig_Result_Bus/1 -> BS_Result/1
  AndN/1 -> result/1, result_tws/1
  BS_Req/1 -> cmp_1/1  "<testSig_RailP_stGrad>"
  BS_Result/1 -> cmp_1/2  "<RailP_stGrad>"
  cmp_1/1 -> tws_1/1, AndN/1
  BS_Req/2 -> cmp_2/1  "<testSig_RailP_bGradMonFinalDef>"
  BS_Result/2 -> cmp_2/2  "<RailP_bGradMonFinalDef>"
  cmp_2/1 -> tws_2/1, AndN/2
  BS_Req/3 -> cmp_3/1  "<testSig_RailP_bGradMonProvDef>"
  BS_Result/3 -> cmp_3/2  "<RailP_bGradMonProvDef>"
  cmp_3/1 -> tws_3/1, AndN/3

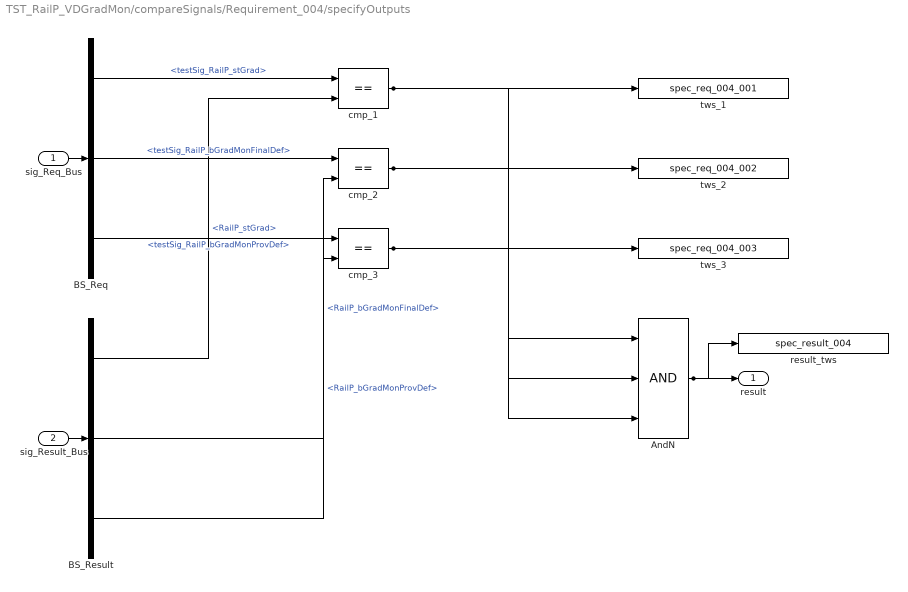
== system TST_RailP_VDGradMon/compareSignals/Requirement_004/specifyOutputs ==
  sig_Req_Bus : Inport
  sig_Result_Bus : Inport  Port=2
  AndN : Logic  Inputs=3
  BS_Req : BusSelector  OutputSignals=testSig_RailP_stGrad,testSig_RailP_bGradMonFinalDef,testSig_RailP_bGradMonProvDef
  BS_Result : BusSelector  OutputSignals=RailP_stGrad,RailP_bGradMonFinalDef,RailP_bGradMonProvDef
  cmp_1 : RelationalOperator  Operator===  RndMeth=Nearest  InputSameDT=on
  cmp_2 : RelationalOperator  Operator===  RndMeth=Nearest  InputSameDT=on
  cmp_3 : RelationalOperator  Operator===  RndMeth=Nearest  InputSameDT=on
  result_tws : ToWorkspace  VariableName=spec_result_004
  tws_1 : ToWorkspace  VariableName=spec_req_004_001
  tws_2 : ToWorkspace  VariableName=spec_req_004_002
  tws_3 : ToWorkspace  VariableName=spec_req_004_003
  result : Outport
  wires:
  sig_Req_Bus/1 -> BS_Req/1
  sig_Result_Bus/1 -> BS_Result/1
  AndN/1 -> result/1, result_tws/1
  BS_Req/1 -> cmp_1/1  "<testSig_RailP_stGrad>"
  BS_Result/1 -> cmp_1/2  "<RailP_stGrad>"
  cmp_1/1 -> tws_1/1, AndN/1
  BS_Req/2 -> cmp_2/1  "<testSig_RailP_bGradMonFinalDef>"
  BS_Result/2 -> cmp_2/2  "<RailP_bGradMonFinalDef>"
  cmp_2/1 -> tws_2/1, AndN/2
  BS_Req/3 -> cmp_3/1  "<testSig_RailP_bGradMonProvDef>"
  BS_Result/3 -> cmp_3/2  "<RailP_bGradMonProvDef>"
  cmp_3/1 -> tws_3/1, AndN/3

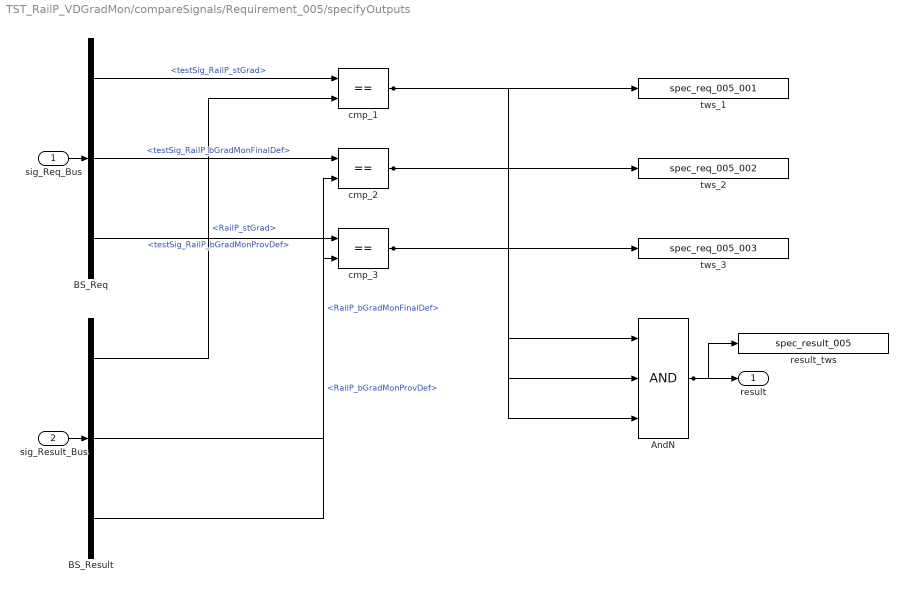
== system TST_RailP_VDGradMon/compareSignals/Requirement_005/specifyOutputs ==
  sig_Req_Bus : Inport
  sig_Result_Bus : Inport  Port=2
  AndN : Logic  Inputs=3
  BS_Req : BusSelector  OutputSignals=testSig_RailP_stGrad,testSig_RailP_bGradMonFinalDef,testSig_RailP_bGradMonProvDef
  BS_Result : BusSelector  OutputSignals=RailP_stGrad,RailP_bGradMonFinalDef,RailP_bGradMonProvDef
  cmp_1 : RelationalOperator  Operator===  RndMeth=Nearest  InputSameDT=on
  cmp_2 : RelationalOperator  Operator===  RndMeth=Nearest  InputSameDT=on
  cmp_3 : RelationalOperator  Operator===  RndMeth=Nearest  InputSameDT=on
  result_tws : ToWorkspace  VariableName=spec_result_005
  tws_1 : ToWorkspace  VariableName=spec_req_005_001
  tws_2 : ToWorkspace  VariableName=spec_req_005_002
  tws_3 : ToWorkspace  VariableName=spec_req_005_003
  result : Outport
  wires:
  sig_Req_Bus/1 -> BS_Req/1
  sig_Result_Bus/1 -> BS_Result/1
  AndN/1 -> result/1, result_tws/1
  BS_Req/1 -> cmp_1/1  "<testSig_RailP_stGrad>"
  BS_Result/1 -> cmp_1/2  "<RailP_stGrad>"
  cmp_1/1 -> tws_1/1, AndN/1
  BS_Req/2 -> cmp_2/1  "<testSig_RailP_bGradMonFinalDef>"
  BS_Result/2 -> cmp_2/2  "<RailP_bGradMonFinalDef>"
  cmp_2/1 -> tws_2/1, AndN/2
  BS_Req/3 -> cmp_3/1  "<testSig_RailP_bGradMonProvDef>"
  BS_Result/3 -> cmp_3/2  "<RailP_bGradMonProvDef>"
  cmp_3/1 -> tws_3/1, AndN/3
